simulink model "ur3_ros2_bridge_v2"  (R2025b)
settings: Solver=VariableStepAuto  StartTime=0.0  StopTime=10.0  RelTol=1e-3
libraries: ros2lib x5
settings Model: Creator=navnoorvirdi  LastModifiedBy=navnoorvirdi

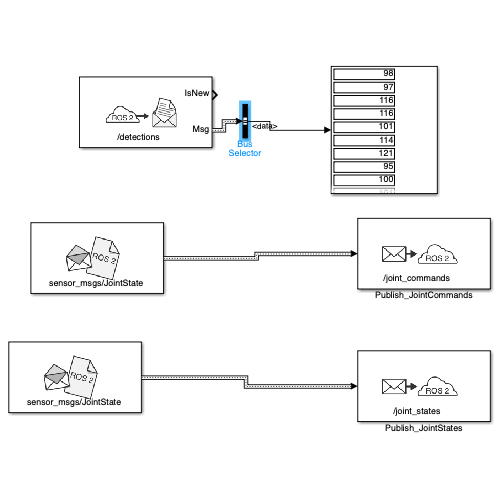
[thumbnail: Simulink's stored preview of the top-level diagram]
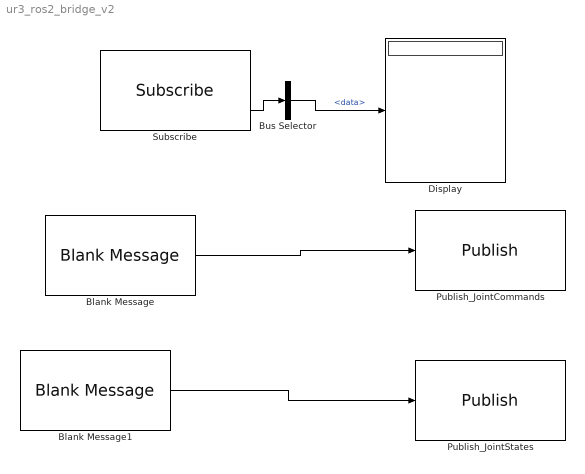
== system ur3_ros2_bridge_v2 ==
  Blank Message : ros2lib/Blank Message  messageClass=Message  entityType=sensor_msgs/JointState  messageType=sensor_msgs/JointState  SampleTime=inf
  Blank Message1 : ros2lib/Blank Message  messageClass=Message  entityType=sensor_msgs/JointState  messageType=sensor_msgs/JointState  SampleTime=inf
  Bus Selector : BusSelector  OutputSignals=data
  Display : Display
  Publish_JointCommands : ros2lib/Publish  topicSource=Select from ROS network  topic=/joint_commands  messageType=sensor_msgs/JointState  QOSHistory=Keep last  QOSDepth=10  QOSReliability=Reliable  QOSDurability=Volatile  QOSDeadline=Inf  QOSLifespan=Inf  QOSLiveliness=Automatic  QOSLeaseDuration=Inf  QOSAvoidROSNamespaceConventions=off
  Publish_JointStates : ros2lib/Publish  topicSource=Specify your own  topic=/joint_states  messageType=sensor_msgs/JointState  QOSHistory=Keep last  QOSDepth=10  QOSReliability=Reliable  QOSDurability=Volatile  QOSDeadline=Inf  QOSLifespan=Inf  QOSLiveliness=Automatic  QOSLeaseDuration=Inf  QOSAvoidROSNamespaceConventions=off
  Subscribe : ros2lib/Subscribe  topicSource=Select from ROS network  topic=/detections  messageType=std_msgs/String  sampleTime=-1  QOSHistory=Keep last  QOSDepth=10  QOSReliability=Reliable  QOSDurability=Volatile  QOSDeadline=Inf  QOSLifespan=Inf  QOSLiveliness=Automatic  QOSLeaseDuration=Inf  QOSAvoidROSNamespaceConventions=off
  wires:
  Subscribe/2 -> Bus Selector/1
  Bus Selector/1 -> Display/1  "<data>"
  Blank Message/1 -> Publish_JointCommands/1
  Blank Message1/1 -> Publish_JointStates/1
